simulink model "simTopLevel"  (R2016b)
settings: Solver=ode15s  StartTime=0.0  StopTime=2  RelTol=1e-3  EnableMultiTasking=on
InitFcn:
  | % minitaurParameters
model workspace (MAT data in the model file):
  MCOS : class17 (value not decoded)
  MCOS : class17 (value not decoded)
  MCOS : class17 (value not decoded)
  MCOS : class17 (value not decoded)
values from neighbouring files (symbols this model uses):
  controlParams = Simulink.Parameter(controlParams)    [minitaurParameters.m]
  envParams = Simulink.Parameter(envParams)    [minitaurParameters.m]
  IC = Simulink.Parameter(IC)    [minitaurParameters.m]
  minitaurParams = Simulink.Parameter(minitaurParams)    [minitaurParameters.m]
undefined symbols (not defined in the file or in its folder): Axis, Fn, ForeRearLag, Period, tau0, tau1, X, Y, Z
libraries: sm_lib x464, fl_lib x132, nesl_utility x41, Contact_Forces_Lib x28, simulink x13, simulink_extras x1
(part 3 of 13)

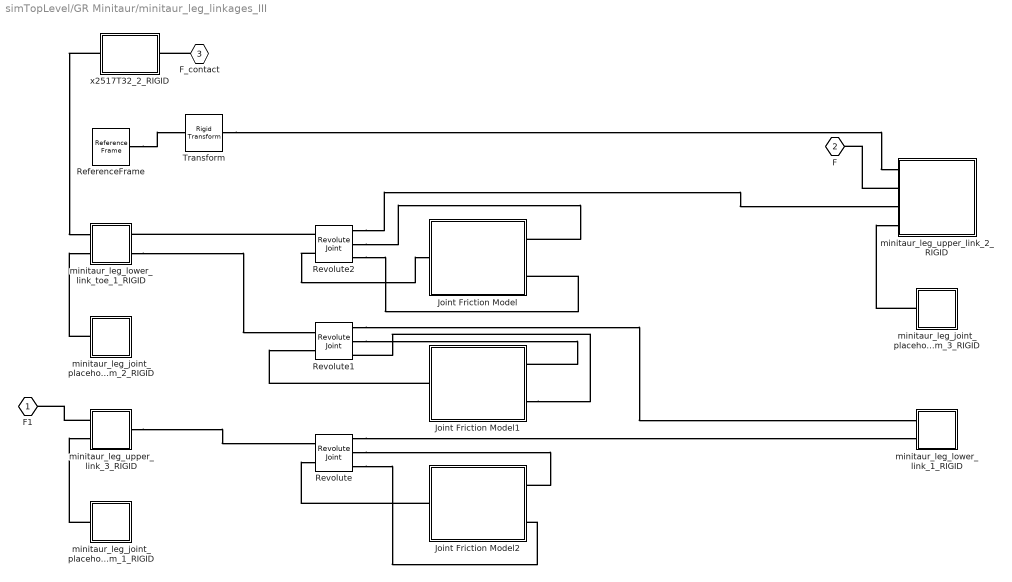
== system simTopLevel/GR Minitaur/minitaur_leg_linkages_III ==
  Joint Friction Model : Subsystem  Variant=on  OverrideUsingVariant=stick-slip  mask(Joint Friction Model){modelVariant=Stick-Slip Friction, leg_joint_radius=minitaurParams.Friction.KneeJoint.EffRadius, linear_region_thresh=minitaurParams.Friction.KneeJoint.VelThresh, mu_k=minitaurParams.Friction.KneeJoint.MuK, mu_s=minitaurParams.Friction.KneeJoint.MuS, fric_bandwidth=minitaurParams.Friction.KneeJoint.FricBandwidth, mu_brk=0, fric_visc_coeff=0, trans_coeff=0}
      mask prompts: modelVariant "Friction Model"; leg_joint_radius "Leg Joint Effective Radius [m]"; linear_region_thresh "Linear Region Velocity Threshold [m/s]"; mu_k "Kinetic Friction Coefficient []"; mu_s "Static Friction Coefficient []"; fric_bandwidth "Friction Model Bandwidth [Hz]"; mu_brk "Breakaway Friction Coefficient []"; fric_visc_coeff "Viscous Friction Coefficient [N*s/m]"; trans_coeff "Transition Approximation Coefficient [s/m]"
      mask help: Models rotational friction present in passive joints. Two options available: stick-slip, and an advanced model that includes viscous and Stribeck friction. Note that in all models, friction is calculated as translational force couple, which is then converted to a friction torque (multiplied by effective joint diameter).
      mask TypeOptions modelVariant: Full Friction | Stick-Slip Friction
      mask Callback modelVariant:
      | currVariant = get_param(gcb,'modelVariant')
      | 
      | switch currVariant
      |     case 'Stick-Slip Friction'
      |         set_param(gcb,'OverrideUsingVariant','stick-slip')
      |         set_param(gcb,'MaskVisibilities',{'on';'on';'on';'on';'on';'on';'off';'off';'off'})
      |     case 'Full Friction'
      |         set_param(gcb,'OverrideUsingVariant','full')
      |         set_param(gcb,'MaskVisibilities',{'on';'on';'on';'on';'off';'off';'on';'on';'on'})
      | 
      | end
  Joint Friction Model1 : Subsystem  Variant=on  OverrideUsingVariant=stick-slip  mask(Joint Friction Model){modelVariant=Stick-Slip Friction, leg_joint_radius=minitaurParams.Friction.KneeJoint.EffRadius, linear_region_thresh=minitaurParams.Friction.KneeJoint.VelThresh, mu_k=minitaurParams.Friction.KneeJoint.MuK, mu_s=minitaurParams.Friction.KneeJoint.MuS, fric_bandwidth=minitaurParams.Friction.KneeJoint.FricBandwidth, mu_brk=0, fric_visc_coeff=0, trans_coeff=0}
      mask prompts: modelVariant "Friction Model"; leg_joint_radius "Leg Joint Effective Radius [m]"; linear_region_thresh "Linear Region Velocity Threshold [m/s]"; mu_k "Kinetic Friction Coefficient []"; mu_s "Static Friction Coefficient []"; fric_bandwidth "Friction Model Bandwidth [Hz]"; mu_brk "Breakaway Friction Coefficient []"; fric_visc_coeff "Viscous Friction Coefficient [N*s/m]"; trans_coeff "Transition Approximation Coefficient [s/m]"
      mask help: Models rotational friction present in passive joints. Two options available: stick-slip, and an advanced model that includes viscous and Stribeck friction. Note that in all models, friction is calculated as translational force couple, which is then converted to a friction torque (multiplied by effective joint diameter).
      mask TypeOptions modelVariant: Full Friction | Stick-Slip Friction
      mask Callback modelVariant:
      | currVariant = get_param(gcb,'modelVariant')
      | 
      | switch currVariant
      |     case 'Stick-Slip Friction'
      |         set_param(gcb,'OverrideUsingVariant','stick-slip')
      |         set_param(gcb,'MaskVisibilities',{'on';'on';'on';'on';'on';'on';'off';'off';'off'})
      |     case 'Full Friction'
      |         set_param(gcb,'OverrideUsingVariant','full')
      |         set_param(gcb,'MaskVisibilities',{'on';'on';'on';'on';'off';'off';'on';'on';'on'})
      | 
      | end
  Joint Friction Model2 : Subsystem  Variant=on  OverrideUsingVariant=stick-slip  mask(Joint Friction Model){modelVariant=Stick-Slip Friction, leg_joint_radius=minitaurParams.Friction.KneeJoint.EffRadius, linear_region_thresh=minitaurParams.Friction.KneeJoint.VelThresh, mu_k=minitaurParams.Friction.KneeJoint.MuK, mu_s=minitaurParams.Friction.KneeJoint.MuS, fric_bandwidth=minitaurParams.Friction.KneeJoint.FricBandwidth, mu_brk=0, fric_visc_coeff=0, trans_coeff=0}
      mask prompts: modelVariant "Friction Model"; leg_joint_radius "Leg Joint Effective Radius [m]"; linear_region_thresh "Linear Region Velocity Threshold [m/s]"; mu_k "Kinetic Friction Coefficient []"; mu_s "Static Friction Coefficient []"; fric_bandwidth "Friction Model Bandwidth [Hz]"; mu_brk "Breakaway Friction Coefficient []"; fric_visc_coeff "Viscous Friction Coefficient [N*s/m]"; trans_coeff "Transition Approximation Coefficient [s/m]"
      mask help: Models rotational friction present in passive joints. Two options available: stick-slip, and an advanced model that includes viscous and Stribeck friction. Note that in all models, friction is calculated as translational force couple, which is then converted to a friction torque (multiplied by effective joint diameter).
      mask TypeOptions modelVariant: Full Friction | Stick-Slip Friction
      mask Callback modelVariant:
      | currVariant = get_param(gcb,'modelVariant')
      | 
      | switch currVariant
      |     case 'Stick-Slip Friction'
      |         set_param(gcb,'OverrideUsingVariant','stick-slip')
      |         set_param(gcb,'MaskVisibilities',{'on';'on';'on';'on';'on';'on';'off';'off';'off'})
      |     case 'Full Friction'
      |         set_param(gcb,'OverrideUsingVariant','full')
      |         set_param(gcb,'MaskVisibilities',{'on';'on';'on';'on';'off';'off';'on';'on';'on'})
      | 
      | end
  ReferenceFrame : sm_lib/Frames and Transforms/Reference Frame
  Revolute : sm_lib/Joints/Revolute Joint  SenseConstraintForce=off  SenseConstraintForceX=off  SenseConstraintForceY=off  SenseConstraintForceZ=off  SenseConstraintTorque=off  SenseConstraintTorqueX=off  SenseConstraintTorqueY=off  SenseConstraintTorqueZ=off  SenseTotalForce=on  SenseTotalForceX=off  SenseTotalForceY=off  SenseTotalForceZ=off  SenseTotalTorque=off  SenseTotalTorqueX=off  SenseTotalTorqueY=off  SenseTotalTorqueZ=off  CompositeWrenchDir=FollowerOnBase  CompositeWrenchFrame=BaseFrame  EquilibriumPosition=0  EquilibriumPositionUnits=rad  SpringStiffness=0  SpringStiffnessUnits=m*N/rad  DampingCoefficient=0  DampingCoefficientUnits=m*s*N/rad  TorqueActuationMode=InputTorque  MotionActuationMode=ComputedMotion  SensePosition=off  SenseVelocity=on  SenseAcceleration=off  SenseTorqueForce=off  PositionTargetSpecify=off  PositionTargetPriority=Low  PositionTargetValue=minitaurParams.RevoluteJoint(1).Rz.Pos  PositionTargetValueUnits=deg  VelocityTargetSpecify=off  VelocityTargetPriority=High  VelocityTargetValue=0  VelocityTargetValueUnits=deg/s
  Revolute1 : sm_lib/Joints/Revolute Joint  SenseConstraintForce=off  SenseConstraintForceX=off  SenseConstraintForceY=off  SenseConstraintForceZ=off  SenseConstraintTorque=off  SenseConstraintTorqueX=off  SenseConstraintTorqueY=off  SenseConstraintTorqueZ=off  SenseTotalForce=on  SenseTotalForceX=off  SenseTotalForceY=off  SenseTotalForceZ=off  SenseTotalTorque=off  SenseTotalTorqueX=off  SenseTotalTorqueY=off  SenseTotalTorqueZ=off  CompositeWrenchDir=FollowerOnBase  CompositeWrenchFrame=BaseFrame  EquilibriumPosition=0  EquilibriumPositionUnits=rad  SpringStiffness=0  SpringStiffnessUnits=m*N/rad  DampingCoefficient=0  DampingCoefficientUnits=m*s*N/rad  TorqueActuationMode=InputTorque  MotionActuationMode=ComputedMotion  SensePosition=off  SenseVelocity=on  SenseAcceleration=off  SenseTorqueForce=off  PositionTargetSpecify=on  PositionTargetPriority=Low  PositionTargetValue=IC.Minitaur.ToeJointL  PositionTargetValueUnits=rad  VelocityTargetSpecify=off  VelocityTargetPriority=High  VelocityTargetValue=0  VelocityTargetValueUnits=deg/s
  Revolute2 : sm_lib/Joints/Revolute Joint  SenseConstraintForce=off  SenseConstraintForceX=off  SenseConstraintForceY=off  SenseConstraintForceZ=off  SenseConstraintTorque=off  SenseConstraintTorqueX=off  SenseConstraintTorqueY=off  SenseConstraintTorqueZ=off  SenseTotalForce=on  SenseTotalForceX=off  SenseTotalForceY=off  SenseTotalForceZ=off  SenseTotalTorque=off  SenseTotalTorqueX=off  SenseTotalTorqueY=off  SenseTotalTorqueZ=off  CompositeWrenchDir=FollowerOnBase  CompositeWrenchFrame=BaseFrame  EquilibriumPosition=0  EquilibriumPositionUnits=rad  SpringStiffness=0  SpringStiffnessUnits=m*N/rad  DampingCoefficient=0  DampingCoefficientUnits=m*s*N/rad  TorqueActuationMode=InputTorque  MotionActuationMode=ComputedMotion  SensePosition=off  SenseVelocity=on  SenseAcceleration=off  SenseTorqueForce=off  PositionTargetSpecify=off  PositionTargetPriority=Low  PositionTargetValue=minitaurParams.RevoluteJoint(3).Rz.Pos  PositionTargetValueUnits=deg  VelocityTargetSpecify=off  VelocityTargetPriority=High  VelocityTargetValue=0  VelocityTargetValueUnits=deg/s
  Transform : sm_lib/Frames and Transforms/Rigid Transform  TranslationMethod=Cartesian  TranslationStandardOffset=0  TranslationLengthUnit=mm  TranslationStandardAxis=+Z  TranslationCartesianOffset=minitaurParams.RigidTransform(16).translation  TranslationROffset=0  TranslationROffsetUnits=m  TranslationZOffset=0  TranslationZOffsetUnits=m  TranslationThetaOffset=0  TranslationThetaOffsetUnits=deg  RotationMethod=ArbitraryAxis  RotationAngleUnits=rad  RotationStandardAxis=+Z  RotationAngle=minitaurParams.RigidTransform(16).angle  RotationArbitraryAxis=minitaurParams.RigidTransform(16).axis  FollAlignAxisA=+X  BaseAlignAxisA=+Y  FollAlignAxisB=+Y  BaseAlignAxisB=+Z  RotationSequenceAxes=FollowerAxes  RotationSequence=XYX  RotationSequenceAngles=[0 0 0]  RotationSequenceAnglesUnits=deg  RotationMatrix=[1 0 0; 0 1 0; 0 0 1]
  minitaur_leg_joint_placeholder_sim_1_RIGID : Subsystem
  minitaur_leg_joint_placeholder_sim_2_RIGID : Subsystem
  minitaur_leg_joint_placeholder_sim_3_RIGID : Subsystem
  minitaur_leg_lower_link_1_RIGID : Subsystem
  minitaur_leg_lower_link_toe_1_RIGID : Subsystem
  minitaur_leg_upper_link_2_RIGID : Subsystem
  minitaur_leg_upper_link_3_RIGID : Subsystem
  x2517T32_2_RIGID : Subsystem
  F1 : PMIOPort  Port=1  Side=Left
  F : PMIOPort  Port=2  Side=Left
  F_contact : PMIOPort  Port=3  Side=Right
  connections:
  minitaur_leg_upper_link_3_RIGID/RConn1 -- Revolute/LConn1
  ReferenceFrame/RConn1 -- Transform/LConn1
  Transform/RConn1 -- minitaur_leg_upper_link_2_RIGID/LConn1
  minitaur_leg_upper_link_2_RIGID/LConn2 -- F/RConn1
  minitaur_leg_upper_link_3_RIGID/LConn1 -- F1/RConn1
  minitaur_leg_lower_link_toe_1_RIGID/RConn2 -- Revolute1/LConn1
  minitaur_leg_joint_placeholder_sim_2_RIGID/LConn1 -- minitaur_leg_lower_link_toe_1_RIGID/LConn2
  Revolute2/LConn1 -- minitaur_leg_lower_link_toe_1_RIGID/RConn1
  x2517T32_2_RIGID/LConn1 -- minitaur_leg_lower_link_toe_1_RIGID/LConn1
  minitaur_leg_joint_placeholder_sim_1_RIGID/LConn1 -- minitaur_leg_upper_link_3_RIGID/LConn2
  minitaur_leg_joint_placeholder_sim_3_RIGID/LConn1 -- minitaur_leg_upper_link_2_RIGID/LConn4
  F_contact/RConn1 -- x2517T32_2_RIGID/RConn1
  Joint Friction Model2/RConn1 -- Revolute/LConn2
  Joint Friction Model1/RConn1 -- Revolute1/LConn2
  Revolute/RConn1 -- minitaur_leg_lower_link_1_RIGID/LConn2
  Revolute2/LConn2 -- Joint Friction Model/RConn1
  Revolute2/RConn1 -- minitaur_leg_upper_link_2_RIGID/LConn3
  Revolute2/RConn3 -- Joint Friction Model/LConn2
  Joint Friction Model1/LConn2 -- Revolute1/RConn3
  Revolute/RConn2 -- Joint Friction Model2/LConn1
  Revolute2/RConn2 -- Joint Friction Model/LConn1
  Revolute/RConn3 -- Joint Friction Model2/LConn2
  Revolute1/RConn2 -- Joint Friction Model1/LConn1
  Revolute1/RConn1 -- minitaur_leg_lower_link_1_RIGID/LConn1

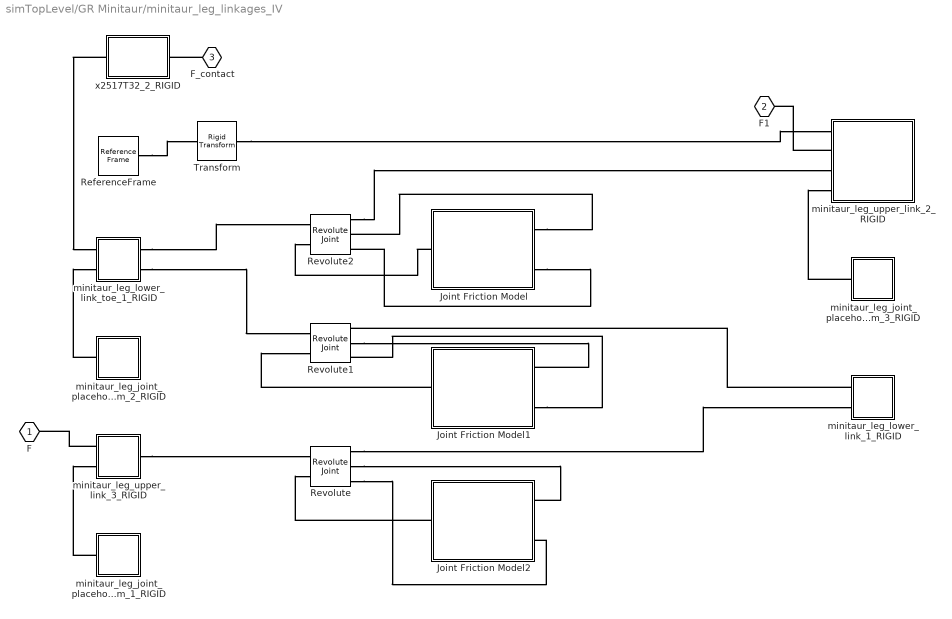
== system simTopLevel/GR Minitaur/minitaur_leg_linkages_IV ==
  Joint Friction Model : Subsystem  Variant=on  OverrideUsingVariant=stick-slip  mask(Joint Friction Model){modelVariant=Stick-Slip Friction, leg_joint_radius=minitaurParams.Friction.KneeJoint.EffRadius, linear_region_thresh=minitaurParams.Friction.KneeJoint.VelThresh, mu_k=minitaurParams.Friction.KneeJoint.MuK, mu_s=minitaurParams.Friction.KneeJoint.MuS, fric_bandwidth=minitaurParams.Friction.KneeJoint.FricBandwidth, mu_brk=0, fric_visc_coeff=0, trans_coeff=0}
      mask prompts: modelVariant "Friction Model"; leg_joint_radius "Leg Joint Effective Radius [m]"; linear_region_thresh "Linear Region Velocity Threshold [m/s]"; mu_k "Kinetic Friction Coefficient []"; mu_s "Static Friction Coefficient []"; fric_bandwidth "Friction Model Bandwidth [Hz]"; mu_brk "Breakaway Friction Coefficient []"; fric_visc_coeff "Viscous Friction Coefficient [N*s/m]"; trans_coeff "Transition Approximation Coefficient [s/m]"
      mask help: Models rotational friction present in passive joints. Two options available: stick-slip, and an advanced model that includes viscous and Stribeck friction. Note that in all models, friction is calculated as translational force couple, which is then converted to a friction torque (multiplied by effective joint diameter).
      mask TypeOptions modelVariant: Full Friction | Stick-Slip Friction
      mask Callback modelVariant:
      | currVariant = get_param(gcb,'modelVariant')
      | 
      | switch currVariant
      |     case 'Stick-Slip Friction'
      |         set_param(gcb,'OverrideUsingVariant','stick-slip')
      |         set_param(gcb,'MaskVisibilities',{'on';'on';'on';'on';'on';'on';'off';'off';'off'})
      |     case 'Full Friction'
      |         set_param(gcb,'OverrideUsingVariant','full')
      |         set_param(gcb,'MaskVisibilities',{'on';'on';'on';'on';'off';'off';'on';'on';'on'})
      | 
      | end
  Joint Friction Model1 : Subsystem  Variant=on  OverrideUsingVariant=stick-slip  mask(Joint Friction Model){modelVariant=Stick-Slip Friction, leg_joint_radius=minitaurParams.Friction.KneeJoint.EffRadius, linear_region_thresh=minitaurParams.Friction.KneeJoint.VelThresh, mu_k=minitaurParams.Friction.KneeJoint.MuK, mu_s=minitaurParams.Friction.KneeJoint.MuS, fric_bandwidth=minitaurParams.Friction.KneeJoint.FricBandwidth, mu_brk=0, fric_visc_coeff=0, trans_coeff=0}
      mask prompts: modelVariant "Friction Model"; leg_joint_radius "Leg Joint Effective Radius [m]"; linear_region_thresh "Linear Region Velocity Threshold [m/s]"; mu_k "Kinetic Friction Coefficient []"; mu_s "Static Friction Coefficient []"; fric_bandwidth "Friction Model Bandwidth [Hz]"; mu_brk "Breakaway Friction Coefficient []"; fric_visc_coeff "Viscous Friction Coefficient [N*s/m]"; trans_coeff "Transition Approximation Coefficient [s/m]"
      mask help: Models rotational friction present in passive joints. Two options available: stick-slip, and an advanced model that includes viscous and Stribeck friction. Note that in all models, friction is calculated as translational force couple, which is then converted to a friction torque (multiplied by effective joint diameter).
      mask TypeOptions modelVariant: Full Friction | Stick-Slip Friction
      mask Callback modelVariant:
      | currVariant = get_param(gcb,'modelVariant')
      | 
      | switch currVariant
      |     case 'Stick-Slip Friction'
      |         set_param(gcb,'OverrideUsingVariant','stick-slip')
      |         set_param(gcb,'MaskVisibilities',{'on';'on';'on';'on';'on';'on';'off';'off';'off'})
      |     case 'Full Friction'
      |         set_param(gcb,'OverrideUsingVariant','full')
      |         set_param(gcb,'MaskVisibilities',{'on';'on';'on';'on';'off';'off';'on';'on';'on'})
      | 
      | end
  Joint Friction Model2 : Subsystem  Variant=on  OverrideUsingVariant=stick-slip  mask(Joint Friction Model){modelVariant=Stick-Slip Friction, leg_joint_radius=minitaurParams.Friction.KneeJoint.EffRadius, linear_region_thresh=minitaurParams.Friction.KneeJoint.VelThresh, mu_k=minitaurParams.Friction.KneeJoint.MuK, mu_s=minitaurParams.Friction.KneeJoint.MuS, fric_bandwidth=minitaurParams.Friction.KneeJoint.FricBandwidth, mu_brk=0, fric_visc_coeff=0, trans_coeff=0}
      mask prompts: modelVariant "Friction Model"; leg_joint_radius "Leg Joint Effective Radius [m]"; linear_region_thresh "Linear Region Velocity Threshold [m/s]"; mu_k "Kinetic Friction Coefficient []"; mu_s "Static Friction Coefficient []"; fric_bandwidth "Friction Model Bandwidth [Hz]"; mu_brk "Breakaway Friction Coefficient []"; fric_visc_coeff "Viscous Friction Coefficient [N*s/m]"; trans_coeff "Transition Approximation Coefficient [s/m]"
      mask help: Models rotational friction present in passive joints. Two options available: stick-slip, and an advanced model that includes viscous and Stribeck friction. Note that in all models, friction is calculated as translational force couple, which is then converted to a friction torque (multiplied by effective joint diameter).
      mask TypeOptions modelVariant: Full Friction | Stick-Slip Friction
      mask Callback modelVariant:
      | currVariant = get_param(gcb,'modelVariant')
      | 
      | switch currVariant
      |     case 'Stick-Slip Friction'
      |         set_param(gcb,'OverrideUsingVariant','stick-slip')
      |         set_param(gcb,'MaskVisibilities',{'on';'on';'on';'on';'on';'on';'off';'off';'off'})
      |     case 'Full Friction'
      |         set_param(gcb,'OverrideUsingVariant','full')
      |         set_param(gcb,'MaskVisibilities',{'on';'on';'on';'on';'off';'off';'on';'on';'on'})
      | 
      | end
  ReferenceFrame : sm_lib/Frames and Transforms/Reference Frame
  Revolute : sm_lib/Joints/Revolute Joint  SenseConstraintForce=off  SenseConstraintForceX=off  SenseConstraintForceY=off  SenseConstraintForceZ=off  SenseConstraintTorque=off  SenseConstraintTorqueX=off  SenseConstraintTorqueY=off  SenseConstraintTorqueZ=off  SenseTotalForce=on  SenseTotalForceX=off  SenseTotalForceY=off  SenseTotalForceZ=off  SenseTotalTorque=off  SenseTotalTorqueX=off  SenseTotalTorqueY=off  SenseTotalTorqueZ=off  CompositeWrenchDir=FollowerOnBase  CompositeWrenchFrame=BaseFrame  EquilibriumPosition=0  EquilibriumPositionUnits=rad  SpringStiffness=0  SpringStiffnessUnits=m*N/rad  DampingCoefficient=0  DampingCoefficientUnits=m*s*N/rad  TorqueActuationMode=InputTorque  MotionActuationMode=ComputedMotion  SensePosition=off  SenseVelocity=on  SenseAcceleration=off  SenseTorqueForce=off  PositionTargetSpecify=off  PositionTargetPriority=Low  PositionTargetValue=minitaurParams.RevoluteJoint(1).Rz.Pos  PositionTargetValueUnits=deg  VelocityTargetSpecify=off  VelocityTargetPriority=High  VelocityTargetValue=0  VelocityTargetValueUnits=deg/s
  Revolute1 : sm_lib/Joints/Revolute Joint  SenseConstraintForce=off  SenseConstraintForceX=off  SenseConstraintForceY=off  SenseConstraintForceZ=off  SenseConstraintTorque=off  SenseConstraintTorqueX=off  SenseConstraintTorqueY=off  SenseConstraintTorqueZ=off  SenseTotalForce=on  SenseTotalForceX=off  SenseTotalForceY=off  SenseTotalForceZ=off  SenseTotalTorque=off  SenseTotalTorqueX=off  SenseTotalTorqueY=off  SenseTotalTorqueZ=off  CompositeWrenchDir=FollowerOnBase  CompositeWrenchFrame=BaseFrame  EquilibriumPosition=0  EquilibriumPositionUnits=rad  SpringStiffness=0  SpringStiffnessUnits=m*N/rad  DampingCoefficient=0  DampingCoefficientUnits=m*s*N/rad  TorqueActuationMode=InputTorque  MotionActuationMode=ComputedMotion  SensePosition=off  SenseVelocity=on  SenseAcceleration=off  SenseTorqueForce=off  PositionTargetSpecify=on  PositionTargetPriority=Low  PositionTargetValue=IC.Minitaur.ToeJointR  PositionTargetValueUnits=rad  VelocityTargetSpecify=off  VelocityTargetPriority=High  VelocityTargetValue=0  VelocityTargetValueUnits=deg/s
  Revolute2 : sm_lib/Joints/Revolute Joint  SenseConstraintForce=off  SenseConstraintForceX=off  SenseConstraintForceY=off  SenseConstraintForceZ=off  SenseConstraintTorque=off  SenseConstraintTorqueX=off  SenseConstraintTorqueY=off  SenseConstraintTorqueZ=off  SenseTotalForce=on  SenseTotalForceX=off  SenseTotalForceY=off  SenseTotalForceZ=off  SenseTotalTorque=off  SenseTotalTorqueX=off  SenseTotalTorqueY=off  SenseTotalTorqueZ=off  CompositeWrenchDir=FollowerOnBase  CompositeWrenchFrame=BaseFrame  EquilibriumPosition=0  EquilibriumPositionUnits=rad  SpringStiffness=0  SpringStiffnessUnits=m*N/rad  DampingCoefficient=0  DampingCoefficientUnits=m*s*N/rad  TorqueActuationMode=InputTorque  MotionActuationMode=ComputedMotion  SensePosition=off  SenseVelocity=on  SenseAcceleration=off  SenseTorqueForce=off  PositionTargetSpecify=off  PositionTargetPriority=Low  PositionTargetValue=minitaurParams.RevoluteJoint(3).Rz.Pos  PositionTargetValueUnits=deg  VelocityTargetSpecify=off  VelocityTargetPriority=High  VelocityTargetValue=0  VelocityTargetValueUnits=deg/s
  Transform : sm_lib/Frames and Transforms/Rigid Transform  TranslationMethod=Cartesian  TranslationStandardOffset=0  TranslationLengthUnit=mm  TranslationStandardAxis=+Z  TranslationCartesianOffset=minitaurParams.RigidTransform(16).translation  TranslationROffset=0  TranslationROffsetUnits=m  TranslationZOffset=0  TranslationZOffsetUnits=m  TranslationThetaOffset=0  TranslationThetaOffsetUnits=deg  RotationMethod=ArbitraryAxis  RotationAngleUnits=rad  RotationStandardAxis=+Z  RotationAngle=minitaurParams.RigidTransform(16).angle  RotationArbitraryAxis=minitaurParams.RigidTransform(16).axis  FollAlignAxisA=+X  BaseAlignAxisA=+Y  FollAlignAxisB=+Y  BaseAlignAxisB=+Z  RotationSequenceAxes=FollowerAxes  RotationSequence=XYX  RotationSequenceAngles=[0 0 0]  RotationSequenceAnglesUnits=deg  RotationMatrix=[1 0 0; 0 1 0; 0 0 1]
  minitaur_leg_joint_placeholder_sim_1_RIGID : Subsystem
  minitaur_leg_joint_placeholder_sim_2_RIGID : Subsystem
  minitaur_leg_joint_placeholder_sim_3_RIGID : Subsystem
  minitaur_leg_lower_link_1_RIGID : Subsystem
  minitaur_leg_lower_link_toe_1_RIGID : Subsystem
  minitaur_leg_upper_link_2_RIGID : Subsystem
  minitaur_leg_upper_link_3_RIGID : Subsystem
  x2517T32_2_RIGID : Subsystem
  F : PMIOPort  Port=1  Side=Left
  F1 : PMIOPort  Port=2  Side=Left
  F_contact : PMIOPort  Port=3  Side=Right
  connections:
  ReferenceFrame/RConn1 -- Transform/LConn1
  Transform/RConn1 -- minitaur_leg_upper_link_2_RIGID/LConn1
  minitaur_leg_upper_link_3_RIGID/LConn1 -- F/RConn1
  minitaur_leg_upper_link_2_RIGID/LConn2 -- F1/RConn1
  minitaur_leg_joint_placeholder_sim_2_RIGID/LConn1 -- minitaur_leg_lower_link_toe_1_RIGID/LConn2
  x2517T32_2_RIGID/LConn1 -- minitaur_leg_lower_link_toe_1_RIGID/LConn1
  minitaur_leg_joint_placeholder_sim_1_RIGID/LConn1 -- minitaur_leg_upper_link_3_RIGID/LConn2
  minitaur_leg_joint_placeholder_sim_3_RIGID/LConn1 -- minitaur_leg_upper_link_2_RIGID/LConn4
  F_contact/RConn1 -- x2517T32_2_RIGID/RConn1
  Joint Friction Model2/RConn1 -- Revolute/LConn2
  Joint Friction Model1/RConn1 -- Revolute1/LConn2
  Revolute/RConn1 -- minitaur_leg_lower_link_1_RIGID/LConn2
  Joint Friction Model/RConn1 -- Revolute2/LConn2
  Revolute2/RConn1 -- minitaur_leg_upper_link_2_RIGID/LConn3
  Joint Friction Model/LConn2 -- Revolute2/RConn3
  Joint Friction Model1/LConn2 -- Revolute1/RConn3
  Revolute/RConn2 -- Joint Friction Model2/LConn1
  Joint Friction Model/LConn1 -- Revolute2/RConn2
  Revolute/RConn3 -- Joint Friction Model2/LConn2
  Revolute1/RConn2 -- Joint Friction Model1/LConn1
  minitaur_leg_lower_link_toe_1_RIGID/RConn1 -- Revolute2/LConn1
  minitaur_leg_lower_link_toe_1_RIGID/RConn2 -- Revolute1/LConn1
  minitaur_leg_upper_link_3_RIGID/RConn1 -- Revolute/LConn1
  minitaur_leg_lower_link_1_RIGID/LConn1 -- Revolute1/RConn1

== system simTopLevel/GR Minitaur/minitaur_motor_module_IA ==
  Desired Torque : Inport
  DYS_BLDC_86x10_BE8108_12 : Subsystem
  Encoder Model : Subsystem  mask{enc_zero=minitaurParams.Sensing.Encoders.IA.Zero}
      mask prompts: enc_zero "Encoder Zero Value [rad]"
  ReferenceFrame : sm_lib/Frames and Transforms/Reference Frame
  Transform : sm_lib/Frames and Transforms/Rigid Transform  TranslationMethod=Cartesian  TranslationStandardOffset=0  TranslationLengthUnit=mm  TranslationStandardAxis=+Z  TranslationCartesianOffset=minitaurParams.RigidTransform(24).translation  TranslationROffset=0  TranslationROffsetUnits=m  TranslationZOffset=0  TranslationZOffsetUnits=m  TranslationThetaOffset=0  TranslationThetaOffsetUnits=deg  RotationMethod=ArbitraryAxis  RotationAngleUnits=rad  RotationStandardAxis=+Z  RotationAngle=minitaurParams.RigidTransform(24).angle  RotationArbitraryAxis=minitaurParams.RigidTransform(24).axis  FollAlignAxisA=+X  BaseAlignAxisA=+Y  FollAlignAxisB=+Y  BaseAlignAxisB=+Z  RotationSequenceAxes=FollowerAxes  RotationSequence=XYX  RotationSequenceAngles=[0 0 0]  RotationSequenceAnglesUnits=deg  RotationMatrix=[1 0 0; 0 1 0; 0 0 1]
  minitaur_motor_driver_board_1_RIGID : Subsystem
  minitaur_motor_driver_cover_1_RIGID : Subsystem
  minitaur_motor_module_plate_1_RIGID : Subsystem
  F1 : PMIOPort  Port=1  Side=Left
  F : PMIOPort  Port=2  Side=Left
  Encoder Value : Outport
  Mech Power : Outport  Port=2
  Input Power : Outport  Port=3
  wires:
  Encoder Model/1(Encoder Value) -> Encoder Value/1
  DYS_BLDC_86x10_BE8108_12/1(Mech Power) -> Mech Power/1
  Desired Torque/1 -> DYS_BLDC_86x10_BE8108_12/1(Desired Torque)
  DYS_BLDC_86x10_BE8108_12/2(Position) -> Encoder Model/1(Motor Position)
  DYS_BLDC_86x10_BE8108_12/3(Input Power) -> Input Power/1
  connections:
  minitaur_motor_driver_cover_1_RIGID/LConn2 -- minitaur_motor_module_plate_1_RIGID/LConn1
  ReferenceFrame/RConn1 -- Transform/LConn1
  Transform/RConn1 -- minitaur_motor_module_plate_1_RIGID/LConn2
  minitaur_motor_module_plate_1_RIGID/LConn3 -- DYS_BLDC_86x10_BE8108_12/LConn1
  minitaur_motor_driver_board_1_RIGID/LConn1 -- minitaur_motor_driver_cover_1_RIGID/LConn1
  DYS_BLDC_86x10_BE8108_12/LConn2 -- F/RConn1
  DYS_BLDC_86x10_BE8108_12/LConn3 -- F1/RConn1

== system simTopLevel/GR Minitaur/minitaur_motor_module_IB ==
  Desired Torque : Inport
  DYS_BLDC_86x10_BE8108_12 : Subsystem
  Encoder Model : Subsystem  mask{enc_zero=minitaurParams.Sensing.Encoders.IB.Zero}
      mask prompts: enc_zero "Encoder Zero Value [rad]"
  ReferenceFrame : sm_lib/Frames and Transforms/Reference Frame
  Transform : sm_lib/Frames and Transforms/Rigid Transform  TranslationMethod=Cartesian  TranslationStandardOffset=0  TranslationLengthUnit=mm  TranslationStandardAxis=+Z  TranslationCartesianOffset=minitaurParams.RigidTransform(24).translation  TranslationROffset=0  TranslationROffsetUnits=m  TranslationZOffset=0  TranslationZOffsetUnits=m  TranslationThetaOffset=0  TranslationThetaOffsetUnits=deg  RotationMethod=ArbitraryAxis  RotationAngleUnits=rad  RotationStandardAxis=+Z  RotationAngle=minitaurParams.RigidTransform(24).angle  RotationArbitraryAxis=minitaurParams.RigidTransform(24).axis  FollAlignAxisA=+X  BaseAlignAxisA=+Y  FollAlignAxisB=+Y  BaseAlignAxisB=+Z  RotationSequenceAxes=FollowerAxes  RotationSequence=XYX  RotationSequenceAngles=[0 0 0]  RotationSequenceAnglesUnits=deg  RotationMatrix=[1 0 0; 0 1 0; 0 0 1]
  minitaur_motor_driver_board_1_RIGID : Subsystem
  minitaur_motor_driver_cover_1_RIGID : Subsystem
  minitaur_motor_module_plate_1_RIGID : Subsystem
  F1 : PMIOPort  Port=1  Side=Left
  F : PMIOPort  Port=2  Side=Left
  Encoder Value : Outport
  Mech Power : Outport  Port=2
  Input Power : Outport  Port=3
  wires:
  Encoder Model/1(Encoder Value) -> Encoder Value/1
  DYS_BLDC_86x10_BE8108_12/1(Mech Power) -> Mech Power/1
  DYS_BLDC_86x10_BE8108_12/2(Position) -> Encoder Model/1(Motor Position)
  Desired Torque/1 -> DYS_BLDC_86x10_BE8108_12/1(Desired Torque)
  DYS_BLDC_86x10_BE8108_12/3(Input Power) -> Input Power/1
  connections:
  minitaur_motor_driver_cover_1_RIGID/LConn2 -- minitaur_motor_module_plate_1_RIGID/LConn1
  ReferenceFrame/RConn1 -- Transform/LConn1
  Transform/RConn1 -- minitaur_motor_module_plate_1_RIGID/LConn2
  DYS_BLDC_86x10_BE8108_12/LConn1 -- minitaur_motor_module_plate_1_RIGID/LConn3
  minitaur_motor_driver_board_1_RIGID/LConn1 -- minitaur_motor_driver_cover_1_RIGID/LConn1
  DYS_BLDC_86x10_BE8108_12/LConn2 -- F/RConn1
  DYS_BLDC_86x10_BE8108_12/LConn3 -- F1/RConn1

== system simTopLevel/GR Minitaur/minitaur_motor_module_IIA ==
  Desired Torque : Inport
  DYS_BLDC_86x10_BE8108_12 : Subsystem
  Encoder Model : Subsystem  mask{enc_zero=minitaurParams.Sensing.Encoders.IIA.Zero}
      mask prompts: enc_zero "Encoder Zero Value [rad]"
  ReferenceFrame : sm_lib/Frames and Transforms/Reference Frame
  Transform : sm_lib/Frames and Transforms/Rigid Transform  TranslationMethod=Cartesian  TranslationStandardOffset=0  TranslationLengthUnit=mm  TranslationStandardAxis=+Z  TranslationCartesianOffset=minitaurParams.RigidTransform(24).translation  TranslationROffset=0  TranslationROffsetUnits=m  TranslationZOffset=0  TranslationZOffsetUnits=m  TranslationThetaOffset=0  TranslationThetaOffsetUnits=deg  RotationMethod=ArbitraryAxis  RotationAngleUnits=rad  RotationStandardAxis=+Z  RotationAngle=minitaurParams.RigidTransform(24).angle  RotationArbitraryAxis=minitaurParams.RigidTransform(24).axis  FollAlignAxisA=+X  BaseAlignAxisA=+Y  FollAlignAxisB=+Y  BaseAlignAxisB=+Z  RotationSequenceAxes=FollowerAxes  RotationSequence=XYX  RotationSequenceAngles=[0 0 0]  RotationSequenceAnglesUnits=deg  RotationMatrix=[1 0 0; 0 1 0; 0 0 1]
  minitaur_motor_driver_board_1_RIGID : Subsystem
  minitaur_motor_driver_cover_1_RIGID : Subsystem
  minitaur_motor_module_plate_1_RIGID : Subsystem
  F1 : PMIOPort  Port=1  Side=Left
  F : PMIOPort  Port=2  Side=Left
  Encoder Value : Outport
  Mech Power : Outport  Port=2
  Input Power : Outport  Port=3
  wires:
  Encoder Model/1(Encoder Value) -> Encoder Value/1
  Desired Torque/1 -> DYS_BLDC_86x10_BE8108_12/1(Desired Torque)
  DYS_BLDC_86x10_BE8108_12/3(Input Power) -> Input Power/1
  DYS_BLDC_86x10_BE8108_12/2(Position) -> Encoder Model/1(Motor Position)
  DYS_BLDC_86x10_BE8108_12/1(Mech Power) -> Mech Power/1
  connections:
  minitaur_motor_driver_cover_1_RIGID/LConn2 -- minitaur_motor_module_plate_1_RIGID/LConn1
  ReferenceFrame/RConn1 -- Transform/LConn1
  Transform/RConn1 -- minitaur_motor_module_plate_1_RIGID/LConn2
  DYS_BLDC_86x10_BE8108_12/LConn1 -- minitaur_motor_module_plate_1_RIGID/LConn3
  minitaur_motor_driver_board_1_RIGID/LConn1 -- minitaur_motor_driver_cover_1_RIGID/LConn1
  DYS_BLDC_86x10_BE8108_12/LConn2 -- F/RConn1
  DYS_BLDC_86x10_BE8108_12/LConn3 -- F1/RConn1

== system simTopLevel/GR Minitaur/minitaur_motor_module_IIB ==
  Desired Torque : Inport
  DYS_BLDC_86x10_BE8108_12 : Subsystem
  Encoder Model : Subsystem  mask{enc_zero=minitaurParams.Sensing.Encoders.IIB.Zero}
      mask prompts: enc_zero "Encoder Zero Value [rad]"
  ReferenceFrame : sm_lib/Frames and Transforms/Reference Frame
  Transform : sm_lib/Frames and Transforms/Rigid Transform  TranslationMethod=Cartesian  TranslationStandardOffset=0  TranslationLengthUnit=mm  TranslationStandardAxis=+Z  TranslationCartesianOffset=minitaurParams.RigidTransform(24).translation  TranslationROffset=0  TranslationROffsetUnits=m  TranslationZOffset=0  TranslationZOffsetUnits=m  TranslationThetaOffset=0  TranslationThetaOffsetUnits=deg  RotationMethod=ArbitraryAxis  RotationAngleUnits=rad  RotationStandardAxis=+Z  RotationAngle=minitaurParams.RigidTransform(24).angle  RotationArbitraryAxis=minitaurParams.RigidTransform(24).axis  FollAlignAxisA=+X  BaseAlignAxisA=+Y  FollAlignAxisB=+Y  BaseAlignAxisB=+Z  RotationSequenceAxes=FollowerAxes  RotationSequence=XYX  RotationSequenceAngles=[0 0 0]  RotationSequenceAnglesUnits=deg  RotationMatrix=[1 0 0; 0 1 0; 0 0 1]
  minitaur_motor_driver_board_1_RIGID : Subsystem
  minitaur_motor_driver_cover_1_RIGID : Subsystem
  minitaur_motor_module_plate_1_RIGID : Subsystem
  F1 : PMIOPort  Port=1  Side=Left
  F : PMIOPort  Port=2  Side=Left
  Encoder Value : Outport
  Mech Power : Outport  Port=2
  Input Power : Outport  Port=3
  wires:
  Encoder Model/1(Encoder Value) -> Encoder Value/1
  DYS_BLDC_86x10_BE8108_12/1(Mech Power) -> Mech Power/1
  DYS_BLDC_86x10_BE8108_12/2(Position) -> Encoder Model/1(Motor Position)
  Desired Torque/1 -> DYS_BLDC_86x10_BE8108_12/1(Desired Torque)
  DYS_BLDC_86x10_BE8108_12/3(Input Power) -> Input Power/1
  connections:
  minitaur_motor_driver_cover_1_RIGID/LConn2 -- minitaur_motor_module_plate_1_RIGID/LConn1
  ReferenceFrame/RConn1 -- Transform/LConn1
  Transform/RConn1 -- minitaur_motor_module_plate_1_RIGID/LConn2
  DYS_BLDC_86x10_BE8108_12/LConn1 -- minitaur_motor_module_plate_1_RIGID/LConn3
  minitaur_motor_driver_board_1_RIGID/LConn1 -- minitaur_motor_driver_cover_1_RIGID/LConn1
  DYS_BLDC_86x10_BE8108_12/LConn2 -- F/RConn1
  DYS_BLDC_86x10_BE8108_12/LConn3 -- F1/RConn1

== system simTopLevel/GR Minitaur/minitaur_motor_module_IIIA ==
  Desired Torque : Inport
  DYS_BLDC_86x10_BE8108_12 : Subsystem
  Encoder Model : Subsystem  mask{enc_zero=minitaurParams.Sensing.Encoders.IIIA.Zero}
      mask prompts: enc_zero "Encoder Zero Value [rad]"
  ReferenceFrame : sm_lib/Frames and Transforms/Reference Frame
  Transform : sm_lib/Frames and Transforms/Rigid Transform  TranslationMethod=Cartesian  TranslationStandardOffset=0  TranslationLengthUnit=mm  TranslationStandardAxis=+Z  TranslationCartesianOffset=minitaurParams.RigidTransform(24).translation  TranslationROffset=0  TranslationROffsetUnits=m  TranslationZOffset=0  TranslationZOffsetUnits=m  TranslationThetaOffset=0  TranslationThetaOffsetUnits=deg  RotationMethod=ArbitraryAxis  RotationAngleUnits=rad  RotationStandardAxis=+Z  RotationAngle=minitaurParams.RigidTransform(24).angle  RotationArbitraryAxis=minitaurParams.RigidTransform(24).axis  FollAlignAxisA=+X  BaseAlignAxisA=+Y  FollAlignAxisB=+Y  BaseAlignAxisB=+Z  RotationSequenceAxes=FollowerAxes  RotationSequence=XYX  RotationSequenceAngles=[0 0 0]  RotationSequenceAnglesUnits=deg  RotationMatrix=[1 0 0; 0 1 0; 0 0 1]
  minitaur_motor_driver_board_1_RIGID : Subsystem
  minitaur_motor_driver_cover_1_RIGID : Subsystem
  minitaur_motor_module_plate_1_RIGID : Subsystem
  F : PMIOPort  Port=1  Side=Left
  F1 : PMIOPort  Port=2  Side=Left
  Encoder Value : Outport
  Mech Power : Outport  Port=2
  Input Power : Outport  Port=3
  wires:
  Encoder Model/1(Encoder Value) -> Encoder Value/1
  DYS_BLDC_86x10_BE8108_12/1(Mech Power) -> Mech Power/1
  DYS_BLDC_86x10_BE8108_12/2(Position) -> Encoder Model/1(Motor Position)
  Desired Torque/1 -> DYS_BLDC_86x10_BE8108_12/1(Desired Torque)
  DYS_BLDC_86x10_BE8108_12/3(Input Power) -> Input Power/1
  connections:
  minitaur_motor_driver_cover_1_RIGID/LConn2 -- minitaur_motor_module_plate_1_RIGID/LConn1
  ReferenceFrame/RConn1 -- Transform/LConn1
  Transform/RConn1 -- minitaur_motor_module_plate_1_RIGID/LConn2
  DYS_BLDC_86x10_BE8108_12/LConn1 -- minitaur_motor_module_plate_1_RIGID/LConn3
  minitaur_motor_driver_board_1_RIGID/LConn1 -- minitaur_motor_driver_cover_1_RIGID/LConn1
  DYS_BLDC_86x10_BE8108_12/LConn2 -- F/RConn1
  DYS_BLDC_86x10_BE8108_12/LConn3 -- F1/RConn1

== system simTopLevel/GR Minitaur/minitaur_motor_module_IIIB ==
  Desired Torque : Inport
  DYS_BLDC_86x10_BE8108_12 : Subsystem
  Encoder Model : Subsystem  mask{enc_zero=minitaurParams.Sensing.Encoders.IIIB.Zero}
      mask prompts: enc_zero "Encoder Zero Value [rad]"
  ReferenceFrame : sm_lib/Frames and Transforms/Reference Frame
  Transform : sm_lib/Frames and Transforms/Rigid Transform  TranslationMethod=Cartesian  TranslationStandardOffset=0  TranslationLengthUnit=mm  TranslationStandardAxis=+Z  TranslationCartesianOffset=minitaurParams.RigidTransform(24).translation  TranslationROffset=0  TranslationROffsetUnits=m  TranslationZOffset=0  TranslationZOffsetUnits=m  TranslationThetaOffset=0  TranslationThetaOffsetUnits=deg  RotationMethod=ArbitraryAxis  RotationAngleUnits=rad  RotationStandardAxis=+Z  RotationAngle=minitaurParams.RigidTransform(24).angle  RotationArbitraryAxis=minitaurParams.RigidTransform(24).axis  FollAlignAxisA=+X  BaseAlignAxisA=+Y  FollAlignAxisB=+Y  BaseAlignAxisB=+Z  RotationSequenceAxes=FollowerAxes  RotationSequence=XYX  RotationSequenceAngles=[0 0 0]  RotationSequenceAnglesUnits=deg  RotationMatrix=[1 0 0; 0 1 0; 0 0 1]
  minitaur_motor_driver_board_1_RIGID : Subsystem
  minitaur_motor_driver_cover_1_RIGID : Subsystem
  minitaur_motor_module_plate_1_RIGID : Subsystem
  F1 : PMIOPort  Port=1  Side=Left
  F : PMIOPort  Port=2  Side=Left
  Encoder Value : Outport
  Mech Power : Outport  Port=2
  Input Power : Outport  Port=3
  wires:
  Encoder Model/1(Encoder Value) -> Encoder Value/1
  Desired Torque/1 -> DYS_BLDC_86x10_BE8108_12/1(Desired Torque)
  DYS_BLDC_86x10_BE8108_12/3(Input Power) -> Input Power/1
  DYS_BLDC_86x10_BE8108_12/2(Position) -> Encoder Model/1(Motor Position)
  DYS_BLDC_86x10_BE8108_12/1(Mech Power) -> Mech Power/1
  connections:
  minitaur_motor_driver_cover_1_RIGID/LConn2 -- minitaur_motor_module_plate_1_RIGID/LConn1
  ReferenceFrame/RConn1 -- Transform/LConn1
  Transform/RConn1 -- minitaur_motor_module_plate_1_RIGID/LConn2
  DYS_BLDC_86x10_BE8108_12/LConn1 -- minitaur_motor_module_plate_1_RIGID/LConn3
  minitaur_motor_driver_board_1_RIGID/LConn1 -- minitaur_motor_driver_cover_1_RIGID/LConn1
  DYS_BLDC_86x10_BE8108_12/LConn2 -- F/RConn1
  DYS_BLDC_86x10_BE8108_12/LConn3 -- F1/RConn1

== system simTopLevel/GR Minitaur/minitaur_motor_module_IVA ==
  Desired Torque : Inport
  DYS_BLDC_86x10_BE8108_12 : Subsystem
  Encoder Model : Subsystem  mask{enc_zero=minitaurParams.Sensing.Encoders.IVA.Zero}
      mask prompts: enc_zero "Encoder Zero Value [rad]"
  ReferenceFrame : sm_lib/Frames and Transforms/Reference Frame
  Transform : sm_lib/Frames and Transforms/Rigid Transform  TranslationMethod=Cartesian  TranslationStandardOffset=0  TranslationLengthUnit=mm  TranslationStandardAxis=+Z  TranslationCartesianOffset=minitaurParams.RigidTransform(24).translation  TranslationROffset=0  TranslationROffsetUnits=m  TranslationZOffset=0  TranslationZOffsetUnits=m  TranslationThetaOffset=0  TranslationThetaOffsetUnits=deg  RotationMethod=ArbitraryAxis  RotationAngleUnits=rad  RotationStandardAxis=+Z  RotationAngle=minitaurParams.RigidTransform(24).angle  RotationArbitraryAxis=minitaurParams.RigidTransform(24).axis  FollAlignAxisA=+X  BaseAlignAxisA=+Y  FollAlignAxisB=+Y  BaseAlignAxisB=+Z  RotationSequenceAxes=FollowerAxes  RotationSequence=XYX  RotationSequenceAngles=[0 0 0]  RotationSequenceAnglesUnits=deg  RotationMatrix=[1 0 0; 0 1 0; 0 0 1]
  minitaur_motor_driver_board_1_RIGID : Subsystem
  minitaur_motor_driver_cover_1_RIGID : Subsystem
  minitaur_motor_module_plate_1_RIGID : Subsystem
  F : PMIOPort  Port=1  Side=Left
  F1 : PMIOPort  Port=2  Side=Left
  Encoder Value : Outport
  Mech Power : Outport  Port=2
  Input Power : Outport  Port=3
  wires:
  Encoder Model/1(Encoder Value) -> Encoder Value/1
  DYS_BLDC_86x10_BE8108_12/1(Mech Power) -> Mech Power/1
  DYS_BLDC_86x10_BE8108_12/2(Position) -> Encoder Model/1(Motor Position)
  Desired Torque/1 -> DYS_BLDC_86x10_BE8108_12/1(Voltage)
  DYS_BLDC_86x10_BE8108_12/3(Input Power) -> Input Power/1
  connections:
  minitaur_motor_driver_cover_1_RIGID/LConn2 -- minitaur_motor_module_plate_1_RIGID/LConn1
  ReferenceFrame/RConn1 -- Transform/LConn1
  Transform/RConn1 -- minitaur_motor_module_plate_1_RIGID/LConn2
  DYS_BLDC_86x10_BE8108_12/LConn1 -- minitaur_motor_module_plate_1_RIGID/LConn3
  minitaur_motor_driver_board_1_RIGID/LConn1 -- minitaur_motor_driver_cover_1_RIGID/LConn1
  DYS_BLDC_86x10_BE8108_12/LConn2 -- F/RConn1
  DYS_BLDC_86x10_BE8108_12/LConn3 -- F1/RConn1

== system simTopLevel/GR Minitaur/minitaur_motor_module_IVB ==
  Desired Torque : Inport
  DYS_BLDC_86x10_BE8108_12 : Subsystem
  Encoder Model : Subsystem  mask{enc_zero=minitaurParams.Sensing.Encoders.IVB.Zero}
      mask prompts: enc_zero "Encoder Zero Value [rad]"
  ReferenceFrame : sm_lib/Frames and Transforms/Reference Frame
  Transform : sm_lib/Frames and Transforms/Rigid Transform  TranslationMethod=Cartesian  TranslationStandardOffset=0  TranslationLengthUnit=mm  TranslationStandardAxis=+Z  TranslationCartesianOffset=minitaurParams.RigidTransform(24).translation  TranslationROffset=0  TranslationROffsetUnits=m  TranslationZOffset=0  TranslationZOffsetUnits=m  TranslationThetaOffset=0  TranslationThetaOffsetUnits=deg  RotationMethod=ArbitraryAxis  RotationAngleUnits=rad  RotationStandardAxis=+Z  RotationAngle=minitaurParams.RigidTransform(24).angle  RotationArbitraryAxis=minitaurParams.RigidTransform(24).axis  FollAlignAxisA=+X  BaseAlignAxisA=+Y  FollAlignAxisB=+Y  BaseAlignAxisB=+Z  RotationSequenceAxes=FollowerAxes  RotationSequence=XYX  RotationSequenceAngles=[0 0 0]  RotationSequenceAnglesUnits=deg  RotationMatrix=[1 0 0; 0 1 0; 0 0 1]
  minitaur_motor_driver_board_1_RIGID : Subsystem
  minitaur_motor_driver_cover_1_RIGID : Subsystem
  minitaur_motor_module_plate_1_RIGID : Subsystem
  F1 : PMIOPort  Port=1  Side=Left
  F : PMIOPort  Port=2  Side=Left
  Encoder Value : Outport
  Mech Power : Outport  Port=2
  Input Power : Outport  Port=3
  wires:
  Encoder Model/1(Encoder Value) -> Encoder Value/1
  Desired Torque/1 -> DYS_BLDC_86x10_BE8108_12/1(Voltage)
  DYS_BLDC_86x10_BE8108_12/1(Mech Power) -> Mech Power/1
  DYS_BLDC_86x10_BE8108_12/2(Position) -> Encoder Model/1(Motor Position)
  DYS_BLDC_86x10_BE8108_12/3(Input Power) -> Input Power/1
  connections:
  minitaur_motor_driver_cover_1_RIGID/LConn2 -- minitaur_motor_module_plate_1_RIGID/LConn1
  ReferenceFrame/RConn1 -- Transform/LConn1
  Transform/RConn1 -- minitaur_motor_module_plate_1_RIGID/LConn2
  DYS_BLDC_86x10_BE8108_12/LConn1 -- minitaur_motor_module_plate_1_RIGID/LConn3
  minitaur_motor_driver_board_1_RIGID/LConn1 -- minitaur_motor_driver_cover_1_RIGID/LConn1
  DYS_BLDC_86x10_BE8108_12/LConn2 -- F/RConn1
  DYS_BLDC_86x10_BE8108_12/LConn3 -- F1/RConn1

== system simTopLevel/Controller/Trajectory Planner/Elliptical Trajectory ==
  time_per_cycle : Inport
  r_0 : Inport  Port=2
  r_x : Inport  Port=3
  r_y : Inport  Port=4
  thetaTilt : Inport  Port=5
  Ellipse Trajectory : MATLAB Function  TreatAsAtomicUnit=on
  Mux : Mux
  Mux1 : Mux
  Polar to Cartesian : simulink_extras/Transformations/Polar to Cartesian  Commented=on
  XY Graph : simulink/Sinks/XY Graph  Commented=on  xmin=-1  xmax=1  ymin=-1  ymax=1  st=-1
  psi : Outport
  L : Outport  Port=2
  wires:
  r_0/1 -> Ellipse Trajectory/1(r0)
  time_per_cycle/1 -> Ellipse Trajectory/2(t)
  r_y/1 -> Ellipse Trajectory/3(ry)
  r_x/1 -> Ellipse Trajectory/4(rx)
  thetaTilt/1 -> Ellipse Trajectory/5(thetaTilt)
  Ellipse Trajectory/5(theta1) -> Polar to Cartesian/2, Mux1/1
  Ellipse Trajectory/1(L1) -> Polar to Cartesian/1, Mux/1
  Ellipse Trajectory/2(L2) -> Mux/2
  Ellipse Trajectory/3(L3) -> Mux/3
  Ellipse Trajectory/4(L4) -> Mux/4
  Ellipse Trajectory/6(theta2) -> Mux1/2
  Ellipse Trajectory/7(theta3) -> Mux1/3
  Ellipse Trajectory/8(theta4) -> Mux1/4
  Mux1/1 -> psi/1
  Mux/1 -> L/1
  Polar to Cartesian/1 -> XY Graph/1
  Polar to Cartesian/2 -> XY Graph/2

== system simTopLevel/Controller/Trajectory Planner/Leg Router ==
  psi : Inport
  L : Inport  Port=2
  Demux : Demux
  Demux1 : Demux
  Mux{,1..3} (4 alike) : Mux  Inputs=2
  leg 1 : Outport
  leg 2 : Outport  Port=2
  leg 3 : Outport  Port=3
  leg 4 : Outport  Port=4
  wires:
  Demux1/1 -> Mux/2
  Mux1/1 -> leg 2/1
  Demux/2 -> Mux1/1
  Demux/1 -> Mux/1
  psi/1 -> Demux/1
  Mux/1 -> leg 1/1
  Demux1/2 -> Mux1/2
  Mux3/1 -> leg 4/1
  Demux/4 -> Mux3/1
  Mux2/1 -> leg 3/1
  L/1 -> Demux1/1
  Demux/3 -> Mux2/1
  Demux1/3 -> Mux2/2
  Demux1/4 -> Mux3/2

== system simTopLevel/Controller/Trajectory Planner/Phase offset ==
  note: Legs:
      | Right Fore
      | Left Fore
      | Left Rear
      | Right Rear
  note: Boolean: left/right in sync (true) or
      | 180* out of phase(false)
  note: Fraction of period that a fore leg
      | lags behind its corresponding rear leg
  fore_lag_in : Inport
  lr_sync : Inport  Port=2
  Add : Sum
  Constant : Constant  Value=[0.5 0 0 0.5]
  Constant1 : Constant  Value=[0 0 1 1]
  Logical Operator : Logic  Operator=NOT  AllPortsSameDT=off  OutDataTypeStr=boolean
  Product : Product
  Product1 : Product
  phase offsets : Outport
  wires:
  fore_lag_in/1 -> Product/1
  Constant1/1 -> Product/2
  lr_sync/1 -> Logical Operator/1
  Constant/1 -> Product1/2
  Product/1 -> Add/1
  Product1/1 -> Add/2
  Add/1 -> phase offsets/1
  Logical Operator/1 -> Product1/1

== system simTopLevel/GR Minitaur/minitaur_chassis_RIGID/control_electronics_1_RIGID ==
  ReferenceFrame : sm_lib/Frames and Transforms/Reference Frame
  Solid : sm_lib/Body Elements/Solid  InertiaType=Custom  Mass=minitaurParams.Solid(24).mass  MassUnits=kg  CenterOfMass=minitaurParams.Solid(24).CoM  CenterOfMassUnits=mm  MomentsOfInertia=minitaurParams.Solid(24).MoI  MomentsOfInertiaUnits=kg*mm^2  ProductsOfInertia=minitaurParams.Solid(24).PoI  ProductsOfInertiaUnits=kg*mm^2  DensityBased=on  Density=1000  DensityUnits=kg/m^3  DoExposeReferenceFrame=on  SerializedFrames=<Frames/>  GraphicType=FromGeometry  MarkerShape=Sphere  MarkerSize=10  GraphicVisPropType=SimpleVisualProperties  GraphicDiffuseColor=minitaurParams.Solid(24).color  GraphicSpecularColor=[0.5 0.5 0.5 1.0]  GraphicAmbientColor=[0.15 0.15 0.15 1.0]  GraphicEmissiveColor=[0.0 0.0 0.0 1.0]  GraphicShininess=75  GraphicOpacity=minitaurParams.Solid(24).opacity  GeometryShape=FromFile  RectangleSize=[1 1]  RectangleSizeUnits=m  BrickDimensions=[1 1 1]  BrickDimensionUnits=m  CylinderRadius=1  CylinderRadiusUnits=m  CylinderLength=1  CylinderLengthUnits=m  SphereRadius=1  SphereRadiusUnits=m  EllipsoidRadii=[1 1 1]  EllipsoidRadiiUnits=m  ExtrusionCrossSection=[1 1; -1 1; -1 -1; 1 -1]  ExtrusionCrossSectionUnits=m  ExtrusionLength=1  ExtrusionLengthUnits=m  PolygonNumSides=3  PolygonOuterRadius=1  PolygonOuterRadiusUnits=m  ExtGeomFileType=STEP  ExtGeomFileName=model\control-electronics_Default_sldprt.STEP  ExtGeomFileUnits=m  RevolutionCrossSection=[1 1; 1 -1; 2 -1; 2 1]  RevolutionCrossSectionUnits=m  RevolutionExtent=Full  RevolutionAngle=180  RevolutionAngleUnits=deg
  F : PMIOPort  Port=1  Side=Left
  connections:
  ReferenceFrame/RConn1 -- Solid/RConn1 -- F/RConn1

== system simTopLevel/GR Minitaur/minitaur_chassis_RIGID/minitaur_battery_holder_1_RIGID ==
  ReferenceFrame : sm_lib/Frames and Transforms/Reference Frame
  Solid : sm_lib/Body Elements/Solid  InertiaType=Custom  Mass=minitaurParams.Solid(11).mass  MassUnits=kg  CenterOfMass=minitaurParams.Solid(11).CoM  CenterOfMassUnits=mm  MomentsOfInertia=minitaurParams.Solid(11).MoI  MomentsOfInertiaUnits=kg*mm^2  ProductsOfInertia=minitaurParams.Solid(11).PoI  ProductsOfInertiaUnits=kg*mm^2  DensityBased=on  Density=1000  DensityUnits=kg/(m^3)  DoExposeReferenceFrame=on  SerializedFrames=<Frames/>  GraphicType=FromGeometry  MarkerShape=Sphere  MarkerSize=10  GraphicVisPropType=SimpleVisualProperties  GraphicDiffuseColor=minitaurParams.Solid(11).color  GraphicSpecularColor=[0.5 0.5 0.5 1.0]  GraphicAmbientColor=[0.15 0.15 0.15 1.0]  GraphicEmissiveColor=[0.0 0.0 0.0 1.0]  GraphicShininess=75  GraphicOpacity=minitaurParams.Solid(11).opacity  GeometryShape=FromFile  RectangleSize=[1 1]  RectangleSizeUnits=m  BrickDimensions=[1 1 1]  BrickDimensionUnits=m  CylinderRadius=1  CylinderRadiusUnits=m  CylinderLength=1  CylinderLengthUnits=m  SphereRadius=1  SphereRadiusUnits=m  EllipsoidRadii=[1 1 1]  EllipsoidRadiiUnits=m  ExtrusionCrossSection=[1 1; -1 1; -1 -1; 1 -1]  ExtrusionCrossSectionUnits=m  ExtrusionLength=1  ExtrusionLengthUnits=m  PolygonNumSides=3  PolygonOuterRadius=1  PolygonOuterRadiusUnits=m  ExtGeomFileType=STEP  ExtGeomFileName=model/minitaur-battery-holder_Default_sldprt.STEP  ExtGeomFileUnits=m  RevolutionCrossSection=[1 1; 1 -1; 2 -1; 2 1]  RevolutionCrossSectionUnits=m  RevolutionExtent=Full  RevolutionAngle=180  RevolutionAngleUnits=deg
  F : PMIOPort  Port=1  Side=Left
  connections:
  ReferenceFrame/RConn1 -- Solid/RConn1 -- F/RConn1
